simulink model "Control_Schematic_6"  (Simulink 8.3)
settings: Solver=FixedStepDiscrete  StartTime=0.0  StopTime=388.546  FixedStep=Ts  RelTol=1e-3
values from neighbouring files (symbols this model uses):
  B = [0 Kappa]'    [StartUp_5.m]    (also in StartUp_6.m)
  b = 156    [StartUp_10_Validation.m]    (also in StartUp_12.m; StartUp_12a.m; StartUp_2.m; StartUp_5.m)
  K1 = .23    (= 0.23)    [StartUp_12.m]    (also in StartUp_12a.m; StartUp_2.m = PolyCon(1,2); StartUp_5.m = 16; StartUp_6.m = 16)
  K2 = .83    (= 0.83)    [StartUp_12.m]    (also in StartUp_12a.m; StartUp_2.m = 0.7; StartUp_5.m = 8; StartUp_6.m = 8)
  Kappa = (1E3/r)/((jw/r)+(m*r*.4))    (= 0.770469447034)    [StartUp_10_Validation.m]    (also in StartUp_12.m; StartUp_12a.m; StartUp_5.m = 0.000542967645047; StartUp_6.m = 0.000542967645047)
  Obz = c2d(Obs,Ts,'tustin')    [StartUp_2.m]    (also in StartUp_5.m; StartUp_6.m)
  P = [L(1,1) L(2,1);L(3,1) L(4,1)]    [StartUp_5.m]    (also in StartUp_6.m; charatioass.m = roots(K))
  R = 50    [StartUp_2.m]    (also in StartUp_5.m; StartUp_6.m)
  Ts = 1/100    (= 0.01)    [StartUp_10_Validation.m]    (also in StartUp_12.m; StartUp_12a.m; StartUp_2.m = 0.001; StartUp_5.m = 0.001)
undefined symbols (not defined in the file or in its folder): DiscIntNeverNeededParam
undefined symbols (not defined in the file): ADAMS_cwd, ADAMS_exec, ADAMS_host, ADAMS_init, ADAMS_inputs, ADAMS_outputs, ADAMS_prefix, ADAMS_static, ADAMS_sysdir
libraries: cstblocks x2, dspinverses x1, simulink x1
(part 2 of 2)

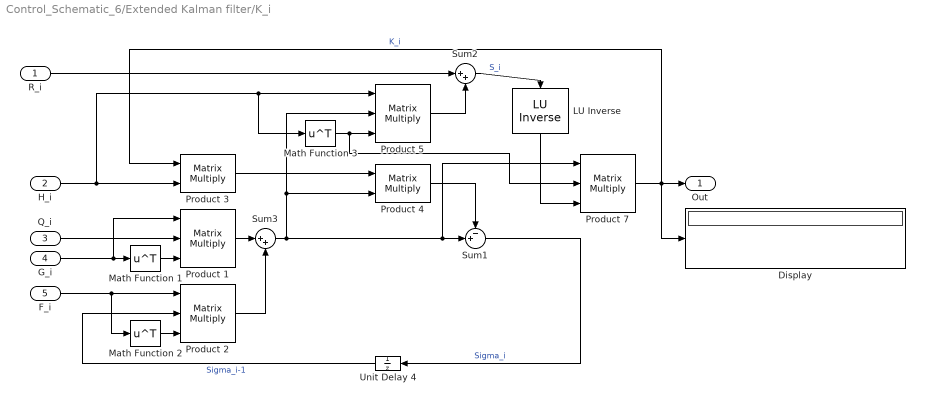
== system Control_Schematic_6/Extended Kalman filter/K_i ==
  R_i : Inport
  H_i : Inport  Port=2
  Q_i : Inport  Port=3
  G_i : Inport  Port=4
  F_i : Inport  Port=5
  " LU Inverse" : dspinverses/ LU Inverse
  Display : Display
  Math Function 1 : Math  Operator=transpose  SaturateOnIntegerOverflow=on
  Math Function 2 : Math  Operator=transpose  SaturateOnIntegerOverflow=on
  Math Function 3 : Math  Operator=transpose  SaturateOnIntegerOverflow=on
  Product {1..2,5,7} (4 alike) : Product  Inputs=3  Multiplication=Matrix(*)
  Product 3 : Product  Multiplication=Matrix(*)
  Product 4 : Product  Multiplication=Matrix(*)
  Sum1 : Sum  Inputs=-+|
  Sum2 : Sum  Inputs=|++
  Sum3 : Sum  Inputs=|++
  Unit Delay 4 : UnitDelay  InitialCondition=[1 0 0;0 1 0;0 0 1]  SampleTime=-1
  Out : Outport
  wires:
  Q_i/1 -> Product 1/2
  G_i/1 -> Math Function 1/1, Product 1/1
  Math Function 1/1 -> Product 1/3
  F_i/1 -> Math Function 2/1, Product 2/1
  Unit Delay 4/1 -> Product 2/2  "Sigma_i-1"
  Math Function 2/1 -> Product 2/3
  Product 1/1 -> Sum3/1
  Product 2/1 -> Sum3/2
  H_i/1 -> Product 5/1, Math Function 3/1, Product 3/2
  Product 7/1 -> Out/1, Display/1, Product 3/1  "K_i"
  Product 3/1 -> Product 4/1
  Sum3/1 -> Product 7/1, Sum1/2, Product 4/2, Product 5/2
  Product 4/1 -> Sum1/1
  Sum1/1 -> Unit Delay 4/1  "Sigma_i"
  Math Function 3/1 -> Product 5/3, Product 7/2
  R_i/1 -> Sum2/1
  Product 5/1 -> Sum2/2
  Sum2/1 -> " LU Inverse"/1  "S_i"
  " LU Inverse"/1 -> Product 7/3

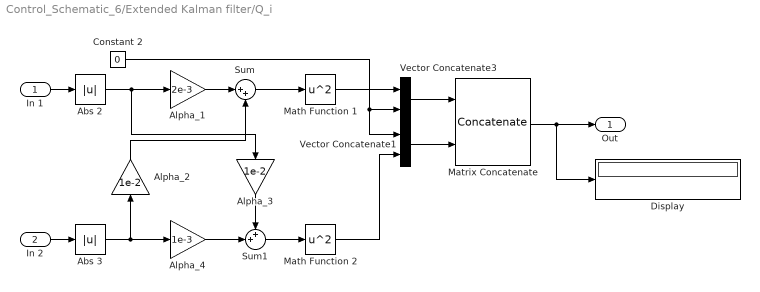
== system Control_Schematic_6/Extended Kalman filter/Q_i ==
  In 1 : Inport
  In 2 : Inport  Port=2
  Abs 2 : Abs
  Abs 3 : Abs
  Alpha_1 : Gain  Gain=2e-3
  Alpha_2 : Gain  Gain=1e-2
  Alpha_3 : Gain  Gain=1e-2
  Alpha_4 : Gain  Gain=1e-3
  Constant 2 : Constant  Value=0
  Display : Display
  Math Function 1 : Math  Operator=square  SaturateOnIntegerOverflow=on
  Math Function 2 : Math  Operator=square  SaturateOnIntegerOverflow=on
  Matrix Concatenate : Concatenate  Mode=Multidimensional array  ConcatenateDimension=2
  Sum : Sum  Inputs=|++
  Sum1 : Sum  Inputs=++|
  Vector Concatenate1 : Concatenate
  Vector Concatenate3 : Concatenate
  Out : Outport
  wires:
  Vector Concatenate1/1 -> Matrix Concatenate/2
  Vector Concatenate3/1 -> Matrix Concatenate/1
  Matrix Concatenate/1 -> Display/1, Out/1
  In 1/1 -> Abs 2/1
  In 2/1 -> Abs 3/1
  Abs 2/1 -> Alpha_3/1, Alpha_1/1
  Abs 3/1 -> Alpha_4/1, Alpha_2/1
  Constant 2/1 -> Vector Concatenate3/2, Vector Concatenate1/1
  Alpha_1/1 -> Sum/1
  Alpha_2/1 -> Sum/2
  Sum/1 -> Math Function 1/1
  Math Function 1/1 -> Vector Concatenate3/1
  Alpha_4/1 -> Sum1/2
  Alpha_3/1 -> Sum1/1
  Sum1/1 -> Math Function 2/1
  Math Function 2/1 -> Vector Concatenate1/2

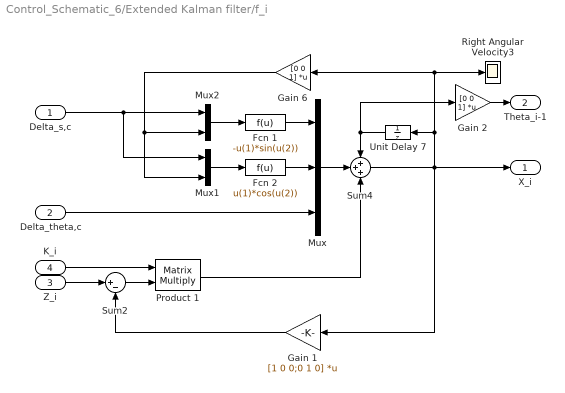
== system Control_Schematic_6/Extended Kalman filter/f_i ==
  Delta_s,c : Inport
  Delta_theta,c : Inport  Port=2
  Z_i : Inport  Port=3
  K_i : Inport  Port=4
  Fcn 1 : Fcn  Expr=-u(1)*sin(u(2))
  Fcn 2 : Fcn  Expr=u(1)*cos(u(2))
  Gain 1 : Gain  Gain=[1 0 0;0 1 0]  Multiplication=Matrix(K*u)
  Gain 2 : Gain  Gain=[0 0 1]  Multiplication=Matrix(K*u)
  Gain 6 : Gain  Gain=[0 0 1]  Multiplication=Matrix(K*u)
  Mux : Mux  Inputs=3
  Mux1 : Mux  Inputs=2
  Mux2 : Mux  Inputs=2
  Product 1 : Product  Multiplication=Matrix(*)
  Right Angular Velocity3 : Scope
      settings: YMin=-1  YMax=1  SaveName=ScopeData30
  Sum2 : Sum  Inputs=|+-
  Sum4 : Sum  Inputs=+++
  Unit Delay 7 : UnitDelay  InitialCondition=[2500 200 0]'  SampleTime=-1
  X_i : Outport
  Theta_i-1 : Outport  Port=2
  wires:
  Mux1/1 -> Fcn 2/1
  Delta_s,c/1 -> Mux1/1, Mux2/1
  Delta_theta,c/1 -> Mux/3
  Mux2/1 -> Fcn 1/1
  Fcn 1/1 -> Mux/1
  Fcn 2/1 -> Mux/2
  Sum4/1 -> X_i/1, Gain 1/1, Unit Delay 7/1, Right Angular Velocity3/1, Gain 6/1
  Gain 6/1 -> Mux1/2, Mux2/2
  Z_i/1 -> Sum2/1
  Gain 1/1 -> Sum2/2
  Sum2/1 -> Product 1/2
  K_i/1 -> Product 1/1
  Unit Delay 7/1 -> Gain 2/1, Sum4/1
  Mux/1 -> Sum4/2
  Product 1/1 -> Sum4/3
  Gain 2/1 -> Theta_i-1/1

== system Control_Schematic_6/Mobile Robot Model/ADAMS Plant ==
  ADAMS inputs : Inport
  S-Function : S-Function  StopFcn=clear mex  FunctionName=adams_plant  Parameters=exevie,exesol,stat,outfil,nampre,o_rate,nam_in,namout,dft,modsim,modani,dt_out,inicmd,exetyp,comtyp,ada_host, workdir,pin_interp_order,pout_extrap_order,pin_extrap_order,pout_interp_order,simulink_lead_cosim  EnableBusSupport=off
  ADAMS outputs : Outport  InitialOutput=0
  wires:
  S-Function/1 -> ADAMS outputs/1
  ADAMS inputs/1 -> S-Function/1

== system Control_Schematic_6/Position reference 1/Clutch 3 ==
  Input : Inport
  Constant1 : Constant
  Digital Clock : DigitalClock  SampleTime=Ts
  Product : Product
  Rear Wheel Angular Speed5 : Scope
      settings: YMin=2.77556e-17  YMax=1  SaveName=ScopeData20
  Sine Wave : Sin  Frequency=(pi/40)  SampleTime=Ts
  Switch : Switch  Threshold=20
  Output : Outport
  wires:
  Constant1/1 -> Switch/1
  Digital Clock/1 -> Switch/2
  Switch/1 -> Rear Wheel Angular Speed5/1, Product/1
  Input/1 -> Product/2
  Product/1 -> Output/1
  Sine Wave/1 -> Switch/3

== system Control_Schematic_6/Position reference 2/Clutch 3 ==
  Input : Inport
  Constant1 : Constant
  Digital Clock : DigitalClock  SampleTime=Ts
  Product : Product
  Rear Wheel Angular Speed5 : Scope
      settings: YMin=2.77556e-17  YMax=1  SaveName=ScopeData20
  Sine Wave : Sin  Frequency=(pi/40)  SampleTime=Ts
  Switch : Switch  Threshold=20
  Output : Outport
  wires:
  Constant1/1 -> Switch/1
  Digital Clock/1 -> Switch/2
  Switch/1 -> Rear Wheel Angular Speed5/1, Product/1
  Input/1 -> Product/2
  Product/1 -> Output/1
  Sine Wave/1 -> Switch/3
